simulink model "SimulacionScara"  (R2019a)
settings: Solver=VariableStepAuto  StartTime=0.0  StopTime=1000.0  RelTol=1e-3
libraries: vrlib x1
settings Model: Creator=HP  LastModifiedBy=HP

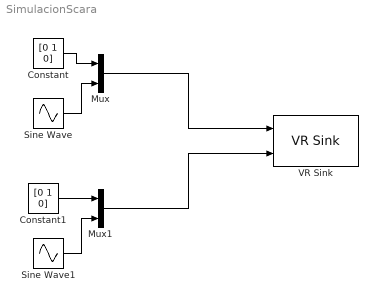
== system SimulacionScara ==
  Constant : Constant  Value=[0 1 0]
  Constant1 : Constant  Value=[0 1 0]
  Mux : Mux  Inputs=2
  Mux1 : Mux  Inputs=2
  Sine Wave : Sin  Amplitude=pi/2  Frequency=0.1  SampleTime=0
  Sine Wave1 : Sin  Amplitude=pi/2  Frequency=0.1  SampleTime=0
  VR Sink : vrlib/VR Sink  InstantiateOnLoad=on  SampleTime=0.1  ViewEnable=on  RemoteChange=off  RemoteView=off  FieldsWritten=Eje1.rotation.4.1.1.double#Eje.rotation.4.1.1.double  WorldFileName=Ensamble.wrl  AutoView=off  VideoDimensions=[]  AllowVariableSize=off  FigureProperties="{'Position', 'Name', 'Viewpoint', 'CameraBound', 'CameraDirection', 'CameraPosition', 'CameraUpVector', 'ZoomFactor', 'Antialiasing', 'Headlight', 'Lighting', 'NavPanel', 'Sound', 'StatusBar', 'Stereo3D', 'Stereo3DCameraOffset', 'Stereo3DHIT', 'ToolBar', 'Textures', 'Transparency', 'Triad', 'Wireframe', 'NavZones', 'NavMode', 'NavSpeed', 'CaptureFileFormat', 'CaptureFileName', 'Record2DCompressMethod', 'Record2DCompressQuality', 'Record2D', 'Record2DFileName', 'Record2DFPS'; [2.0000000000000000e+00   8.4000000000000000e+01   6.8100000000000000e+02   5.9200000000000000e+02], '', '', 'on', [-4.3169273216519471e-01  -2.1767620422425363e-03   9.0201809666035049e-01], [3.9784952883026627e+01   1.5007693052009177e+01  -6.5802484472761648e+01], [-2.3902736319510853e-02   9.9967353225470523e-01  -9.0270762621000866e-03], [1.0000000000000000e+00], 'on', 'on', 'on', 'halfbar', 'on', 'on', 'off', [1.0000000149011612e-01], [0.0000000000000000e+00], 'on', 'on', 'on', 'none', 'off', 'off', 'fly', 'normal', 'tif', '%f_anim_%n.tif', 'auto', [7.5000000000000000e+01], 'off', '%f_anim_%n.avi', 'auto'}"
      settings: SourceProductName=Simulink
  wires:
  Constant/1 -> Mux/1
  Sine Wave/1 -> Mux/2
  Mux/1 -> VR Sink/1
  Constant1/1 -> Mux1/1
  Sine Wave1/1 -> Mux1/2
  Mux1/1 -> VR Sink/2
